simulink model "CtrlSyst_Comp2"  (R2018b)
settings: Solver=FixedStepAuto  StartTime=0.0  StopTime=50  FixedStep=0.0001  RelTol=1e-3
libraries: cstblocks x3
settings Model: Creator=user  LastModifiedBy=NTU
settings DebuggingCC: LibraryContextMissingDiagnostic=none
settings SFSimCC: SimUseLocalCustomCode=off
settings RTWCC: RTWUseLocalCustomCode=off

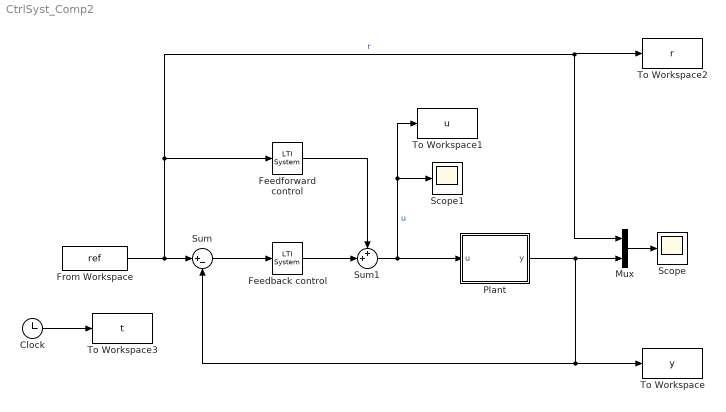
== system CtrlSyst_Comp2 ==
  Clock : Clock
  Feedback control : cstblocks/LTI System  sys=C  IC=[]
  Feedforward control : cstblocks/LTI System  sys=F  IC=[]
  From Workspace : FromWorkspace  VariableName=ref  SampleTime=0
  Mux : Mux  Inputs=2
  Plant : Subsystem
  Scope : Scope
  Scope1 : Scope
  Sum : Sum  Inputs=|+-
  Sum1 : Sum  Inputs=++|
  To Workspace : ToWorkspace  VariableName=y  SampleTime=-1
  To Workspace1 : ToWorkspace  VariableName=u  SampleTime=-1
  To Workspace2 : ToWorkspace  VariableName=r  SampleTime=-1
      settings: Save2DSignal=2-D array (concatenate along first dimension)
  To Workspace3 : ToWorkspace  VariableName=t  SampleTime=-1
  wires:
  From Workspace/1 -> Feedforward control/1, Mux/1, To Workspace2/1, Sum/1  "r"
  Mux/1 -> Scope/1
  Sum1/1 -> To Workspace1/1, Scope1/1, Plant/1(u)  "u"
  Feedforward control/1 -> Sum1/1
  Plant/1(y) -> Sum/2, To Workspace/1, Mux/2
  Clock/1 -> To Workspace3/1
  Sum/1 -> Feedback control/1
  Feedback control/1 -> Sum1/2

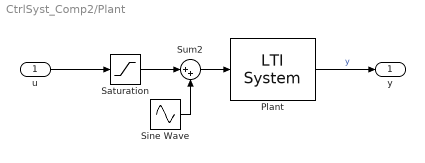
== system CtrlSyst_Comp2/Plant ==
  u : Inport
  Plant : cstblocks/LTI System  sys=P  IC=[]
  Saturation : Saturate  UpperLimit=200  LowerLimit=-200
  Sine Wave : Sin  Amplitude=0.1  Frequency=2.5  SampleTime=0
  Sum2 : Sum  Inputs=|++
  y : Outport
  wires:
  Sine Wave/1 -> Sum2/2
  Plant/1 -> y/1  "y"
  u/1 -> Saturation/1
  Sum2/1 -> Plant/1
  Saturation/1 -> Sum2/1
